simulink model "is95revchdetection2"  (Simulink 4.00)
settings: Solver=VariableStepDiscrete  SolverMode=SingleTasking  StartTime=0.0  StopTime=2  RelTol=1e-3  AbsTol=1e-6
undefined symbols (not defined in the file): slcm
libraries: cdmaprivate x4, cdmalibv1p1 x3, dspsigops x3, commchan2 x2, dspsigattribs x1, commsink2 x1
settings Model: CovMetricSettings=d  Creator=rkumar  LastModifiedBy=akansal  SaveTime=off  SaveOutput=off  LimitDataPoints=off  ExtModeTrigMode=oneshot  ExtModeArmWhenConnect=off  BlockReductionOpt=off

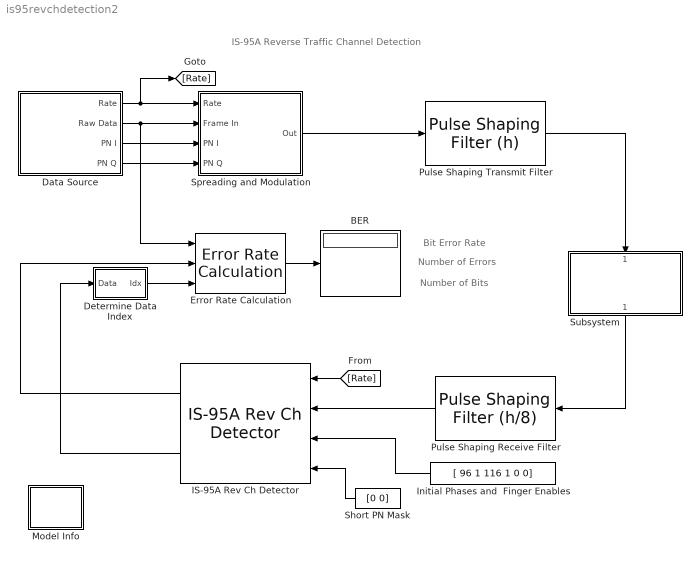
== system is95revchdetection2 ==
  note: IS-95A Reverse Traffic Channel Detection
  note: Bit Error Rate
  note: Number of Errors
  note: Number of Bits
  " Spreading and Modulation " : Subsystem
      settings: RTWFcnNameOpts=Auto  RTWFileNameOpts=Auto
  BER : Display
      settings: Format=short
  Data Source : Subsystem
      settings: RTWFcnNameOpts=Auto  RTWFileNameOpts=Auto
  Determine Data Index : Subsystem
      settings: RTWFcnNameOpts=Auto  RTWFileNameOpts=Auto
  Error Rate Calculation : commsink2/Error Rate Calculation  N=2*576  st_delay=2*576  cp_mode=Select samples from port  subframe=[]  PMode=Port  WsName=ErrorVec  RsMode2=off
  IS-95A Rev Ch Detector : cdmalibv1p1/IS-95A Base Station Receiver/IS-95A Rev Ch Detector  Orientation=left  chType=Traffic  wlshOrd=6  lngcd_mask=1  overSamplRate=8  sampTime=1/(50*384)
  Initial Phases and  Finger Enables : Constant  Orientation=left  Value=[ 96 1 116 1 0 0]
  Model Info : Subsystem  LoadFcn=slcm LoadBlock;  InitFcn=slcm('UpdateAllCMBlocksInThisModelInit')  mask(CMBlock){InitialSaveTempField=, InitialBlockCM=none, BlockCM=none, Frame=on, SaveTempField=, DisplayStringWithTags=Info, MaskDisplayString=Info, HorizontalTextAlignment=Center, LeftAlignmentValue=0.5, SourceBlockDiagram=is95revchdetection2, TagMaxNumber=20, CMTag1=, CMTag2=, CMTag3=, CMTag4=, CMTag5=, CMTag6=, CMTag7=, CMTag8=, CMTag9=, CMTag10=, CMTag11=, CMTag12=, CMTag13=, CMTag14=, CMTag15=, CMTag16=, CMTag17=, CMTag18=, CMTag19=, CMTag20=}
      mask help: This block allows revision control information to be displayed within the model.
      settings: CopyFcn=slcm CopyBlock;  DeleteFcn=slcm Cancel;  PostSaveFcn=slcm('UpdateAllCMBlocksInThisModel')  NameChangeFcn=slcm Rename;  OpenFcn=cdmademohelp;  RTWFcnNameOpts=Auto  RTWFileNameOpts=Auto
      mask Display: text(str2num(LeftAlignmentValue), 0.5, MaskDisplayString, 'HorizontalAlignment', HorizontalTextAlignment)
  Pulse Shaping Receive Filter : cdmaprivate/Pulse Shaping Filter (h//8)  Orientation=left  N=1
  Pulse Shaping Transmit Filter : cdmaprivate/Pulse Shaping Filter (h)  N=1
  Short PN Mask : Constant  Orientation=left  Value=[0 0]
  Subsystem : Subsystem  Orientation=down
      settings: RTWFcnNameOpts=Auto  RTWFileNameOpts=Auto
      mask Display: disp('Rayleigh Multipath\n and  AWGN\nChannel')
  wires:
  " Spreading and Modulation "/1("Out ") -> Pulse Shaping Transmit Filter/1
  Pulse Shaping Transmit Filter/1 -> Subsystem/1(" ")
  Data Source/3(PN I) -> " Spreading and Modulation "/3(PN I)
  Data Source/4(PN Q) -> " Spreading and Modulation "/4(PN Q)
  Data Source/1(Rate) -> " Spreading and Modulation "/1(Rate), [Rate]
  Subsystem/1("  ") -> Pulse Shaping Receive Filter/1
  Short PN Mask/1 -> IS-95A Rev Ch Detector/4
  [Rate] -> IS-95A Rev Ch Detector/1
  Pulse Shaping Receive Filter/1 -> IS-95A Rev Ch Detector/2
  Initial Phases and  Finger Enables/1 -> IS-95A Rev Ch Detector/3
  Determine Data Index/1(Idx) -> Error Rate Calculation/3
  Error Rate Calculation/1 -> BER/1
  IS-95A Rev Ch Detector/2 -> Determine Data Index/1(Data)
  IS-95A Rev Ch Detector/1 -> Error Rate Calculation/2
  Data Source/2(Raw Data) -> " Spreading and Modulation "/2(Frame In), Error Rate Calculation/1

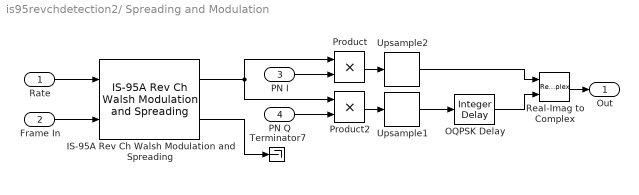
== system is95revchdetection2/ Spreading and Modulation  ==
  Rate : Inport  Port=1
  Frame In : Inport  Port=2
  PN I : Inport  Port=3
  PN Q : Inport  Port=4
  IS-95A Rev Ch Walsh Modulation and Spreading : cdmalibv1p1/IS-95A Mobile Station Transmitter/IS-95A Rev Ch Walsh Modulation and Spreading  chType=Traffic  lngCdMask=1  wlshOrd=6  sampTime=1/(50*384)
  OQPSK Delay : dspsigops/Integer Delay  delay=4  ic=0
  Product : Product  Inputs=2  Multiplication=Element-wise(.*)  SaturateOnIntegerOverflow=on
  Product2 : Product  Inputs=2  Multiplication=Element-wise(.*)  SaturateOnIntegerOverflow=on
  Real-Imag to Complex : RealImagToComplex  Input=RealAndImag  ConstantPart=0
  Terminator7 : Terminator
  Upsample1 : dspsigops/Upsample  N=8  phase=0  ic=0  mode=Maintain input frame rate
  Upsample2 : dspsigops/Upsample  N=8  phase=0  ic=0  mode=Maintain input frame rate
  "Out " : Outport  Port=1
  wires:
  IS-95A Rev Ch Walsh Modulation and Spreading/1 -> Product/1, Product2/1
  Rate/1 -> IS-95A Rev Ch Walsh Modulation and Spreading/1
  PN I/1 -> Product/2
  Frame In/1 -> IS-95A Rev Ch Walsh Modulation and Spreading/2
  PN Q/1 -> Product2/2
  Product/1 -> Upsample2/1
  Product2/1 -> Upsample1/1
  Upsample1/1 -> OQPSK Delay/1
  OQPSK Delay/1 -> Real-Imag to Complex/2
  Upsample2/1 -> Real-Imag to Complex/1
  Real-Imag to Complex/1 -> "Out "/1
  IS-95A Rev Ch Walsh Modulation and Spreading/2 -> Terminator7/1

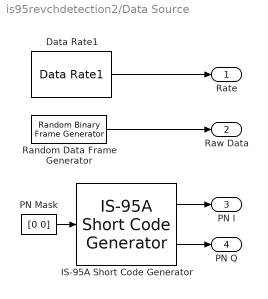
== system is95revchdetection2/Data Source ==
  Data Rate1 : cdmaprivate/Data Rate1  rate=Full
  IS-95A Short Code Generator : cdmalibv1p1/IS-95A Common/IS-95A Short Code Generator  numOut=64  sampTime=1/(50*384)
  PN Mask : Constant  Value=[0 0]
  Random Data Frame Generator : cdmaprivate/Random Binary Frame Generator  seed=119940  Ts=1/(50*576)  N=576
  Rate : Outport  Port=1  InitialOutput=0
  Raw Data : Outport  Port=2  InitialOutput=0
  PN I : Outport  Port=3  InitialOutput=0
  PN Q : Outport  Port=4  InitialOutput=0
  wires:
  Data Rate1/1 -> Rate/1
  PN Mask/1 -> IS-95A Short Code Generator/1
  Random Data Frame Generator/1 -> Raw Data/1
  IS-95A Short Code Generator/1 -> PN I/1
  IS-95A Short Code Generator/2 -> PN Q/1

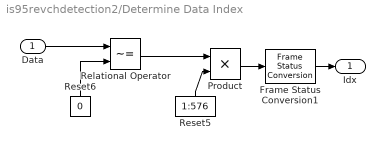
== system is95revchdetection2/Determine Data Index ==
  Data : Inport  Port=1
  Frame Status Conversion1 : dspsigattribs/Frame Status Conversion  growRefPort=off  outframe=Sample-based
  Product : Product  Inputs=2  Multiplication=Element-wise(.*)  SaturateOnIntegerOverflow=on
  Relational Operator : RelationalOperator  Operator=~=
  Reset5 : Constant  Orientation=up  Value=1:576
  Reset6 : Constant  Orientation=up  Value=0
  Idx : Outport  Port=1
  wires:
  Reset6/1 -> Relational Operator/2
  Relational Operator/1 -> Product/1
  Reset5/1 -> Product/2
  Data/1 -> Relational Operator/1
  Product/1 -> Frame Status Conversion1/1
  Frame Status Conversion1/1 -> Idx/1

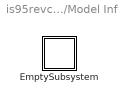
== system is95revchdetection2/Model Info ==
  EmptySubsystem : Subsystem
      settings: RTWFcnNameOpts=Auto  RTWFileNameOpts=Auto

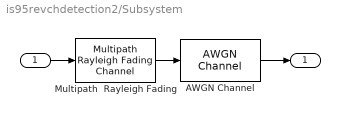
== system is95revchdetection2/Subsystem ==
  " " : Inport  Port=1
  AWGN Channel : commchan2/AWGN Channel  seed=123456  noiseMode="Signal to noise ratio  (Es/No)"  EsNodB=10  SNRdB=10  Ps=1  Tsym=1/1228800  variance=1
  "Multipath  Rayleigh Fading " : commchan2/Multipath Rayleigh Fading Channel  Fd=14.07  simTs=1/(1228800*8)  delayVec=[0 2e-6]  gainVecdB=[0 0]  normGain=on  Seed=831029
  "  " : Outport  Port=1
  wires:
  " "/1 -> "Multipath  Rayleigh Fading "/1
  AWGN Channel/1 -> "  "/1
  "Multipath  Rayleigh Fading "/1 -> AWGN Channel/1

== system is95revchdetection2/Model Info/EmptySubsystem ==
